simulink model "seesaw_quick_start"  (Simulink 7.8)
settings: Solver=ode1  StartTime=0.0  StopTime=inf  FixedStep=0.002  RelTol=1e-3
PostLoadFcn:
  | qc_set_target_type(getConfigSet(bdroot, 'QUARC Default Target Configuration'));
undefined symbols (not defined in the file): HIL
libraries: quarc_library x4, simulink x1
settings Model: Creator=pmartin  LastModifiedBy=pmartin  SimulationMode=external  ExtModeTrigDuration=5000
settings SolverCC: PositivePriorityOrder=on
settings OptimizationCC: InitFltsAndDblsToZero=on
settings DebuggingCC: SaveWithParameterizedLinksMsg=none  MultiTaskDSMMsg=warning  MultiTaskCondExecSysMsg=none  FcnCallInpInsideContextMsg=Use local settings  StrictBusMsg=None
settings RTWCC: SystemTargetFile=quarc_windows.tlc  TemplateMakefile=quarc_default_tmf  Description=QUARC Win32 Target  ProcessScript=quarc_windows_make_rtw_hook
settings STFCustomTargetCC: TargetPreCompLibLocation=C:\PROGRA~2\QUARC\lib\2012b\windows\release  CombineOutputUpdateFcns=on  SystemTargetFile=quarc_windows.tlc
settings GRTTargetCC: TargetPreCompLibLocation=C:\PROGRA~2\QUARC\lib\2012b\windows\release  ParMdlRefBuildCompliant=off  CompOptLevelCompliant=off  ConcurrentExecutionCompliant=off  CombineOutputUpdateFcns=on  MatFileLogging=off  ExtMode=on  ExtModeMexFile=quarc_comm

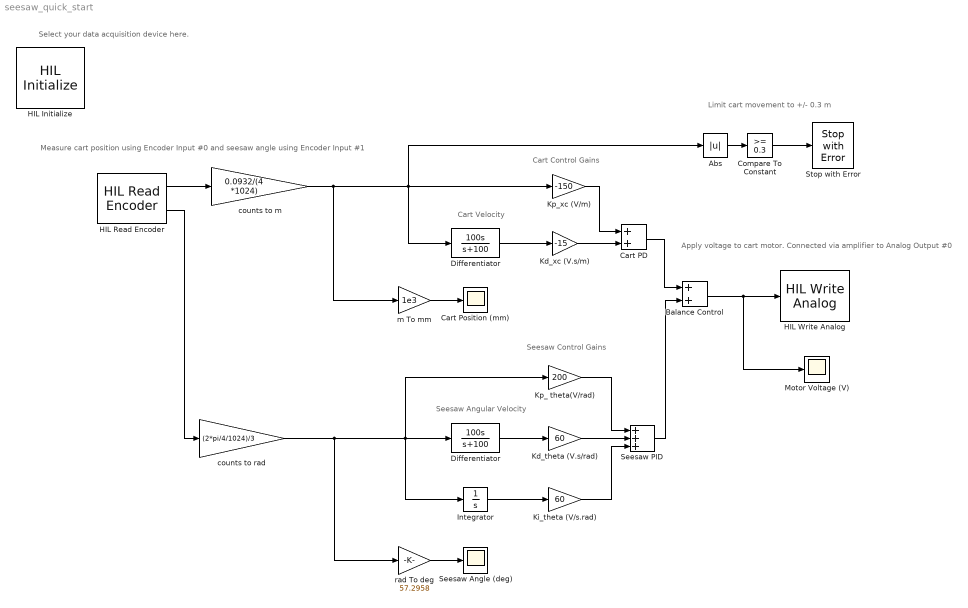
== system seesaw_quick_start ==
  note: Measure cart position using Encoder Input #0
      | and seesaw angle using Encoder Input #1
  note: Select your data acquisition device here.
  note: Cart Control Gains
  note: Cart Velocity
  note: Seesaw Angular Velocity
  note: Seesaw Control Gains
  note: Limit cart movement to +/- 0.3 m
  note: Apply voltage to cart motor.
      | Connected via amplifier to Analog Output #0
  Abs : Abs
  Balance Control : Sum
  Cart PD : Sum
  Cart Position (mm) : Scope
      settings: TickLabels=on  TimeRange=5  YMin=-25  YMax=25  SaveName=data_xc
  Compare To Constant : simulink/Logic and Bit Operations/Compare To Constant  relop=>=  const=0.3  OutDataTypeStr=boolean
  Differentiator : TransferFcn  Numerator=[100 0]  Denominator=[1 100]
  "Differentiator " : TransferFcn  Numerator=[100 0]  Denominator=[1 100]
  HIL Initialize : quarc_library/Data Acquisition/Generic/Configuration/HIL Initialize  object_name=HIL-1  board_type=q2_usb  board_number=0  board_options=d0=digital;d1=digital;led=auto;update_rate=normal  exclusive=off  active=off  hardware_clocks=[0:2]  clock_modes=[]  initial_clock_frequencies=[]  set_clock_params_at_start=off  set_clock_params_at_switch_in=off  set_clock_frequencies_at_start=off  set_clock_frequencies_at_switch_in=off  analog_input_channels=[0:1]  analog_input_maximums=10  analog_input_minimums=-10  set_analog_input_params_at_start=on  set_analog_input_params_at_switch_in=off  analog_output_channels=[0:1]  analog_output_maximums=10  analog_output_minimums=-10  initial_analog_outputs=[0]  final_analog_outputs=[0]  watchdog_analog_outputs=0  set_analog_output_params_at_start=on  set_analog_output_params_at_switch_in=off  set_analog_outputs_at_start=on  set_analog_outputs_at_switch_in=off  set_analog_outputs_at_terminate=on  set_analog_outputs_at_switch_out=off  set_analog_outputs_on_watchdog=off  digital_input_channels=[]  digital_output_channels=[0:7]  digital_output_configuration=[]  initial_digital_outputs=[0]  final_digital_outputs=[0]  watchdog_digital_outputs=[0]  set_digital_output_params_at_start=off  set_digital_output_params_at_switch_in=off  set_digital_outputs_at_start=on  set_digital_outputs_at_switch_in=off  set_digital_outputs_at_terminate=on  set_digital_outputs_at_switch_out=off  set_digital_outputs_on_watchdog=off  encoder_channels=[0:1]  quadrature=[4]  encoder_filter_frequency=[]  initial_encoder_counts=[0]  set_encoder_params_at_start=on  set_encoder_params_at_switch_in=off  set_encoder_counts_at_start=on  set_encoder_counts_at_switch_in=off  pwm_channels=[]  pwm_modes=[0]  pwm_frequency=1/0.020  pwm_configuration=[]  pwm_alignment=[]  pwm_polarity=[]  pwm_leading_deadband=[]  pwm_trailing_deadband=[]  initial_pwm_outputs=[0]  final_pwm_outputs=[0]  watchdog_pwm_outputs=[0]  set_pwm_params_at_start=on  set_pwm_params_at_switch_in=off  set_pwm_outputs_at_start=on  set_pwm_outputs_at_switch_in=off  set_pwm_outputs_at_terminate=on  set_pwm_outputs_at_switch_out=off  set_pwm_outputs_on_watchdog=off  other_output_channels=[]  initial_other_outputs=[]  final_other_outputs=[]  watchdog_other_outputs=[]  set_other_outputs_at_start=off  set_other_outputs_at_switch_in=off  set_other_outputs_at_terminate=off  set_other_outputs_at_switch_out=off  set_other_outputs_on_watchdog=off
  HIL Read Encoder : quarc_library/Data Acquisition/Generic/Immediate I//O/HIL Read Encoder  object_name=HIL-1  channels=[0:1]  sample_time=qc_get_step_size  active=on  vector_output=off  data_type_mode=Inherit via back propagation  data_type=double
  HIL Write Analog : quarc_library/Data Acquisition/Generic/Immediate I//O/HIL Write Analog  object_name=HIL-1  channels=0  sample_time=-1  active=off  vector_input=off
  Integrator : Integrator
  Kd_theta (V.s/rad) : Gain  Gain=60
  Kd_xc (V.s/m) : Gain  Gain=-15
  Ki_theta (V/s.rad) : Gain  Gain=60
  Kp_ theta(V/rad) : Gain  Gain=200
  Kp_xc (V/m) : Gain  Gain=-150
  Motor Voltage (V) : Scope
  Seesaw Angle (deg) : Scope
      settings: TimeRange=5  YMin=-32.5  YMax=32.5  SaveName=data_xjc
  Seesaw PID : Sum  Inputs=+++
  Stop with Error : quarc_library/Sinks/Error Handling/Stop with Error  message_type=Fixed error message  message=Cart position limit reached
      settings: AttributesFormatString="\"%<message>\""
  counts to m : Gain  Gain=0.0932/(4 *1024)  SaturateOnIntegerOverflow=on  OutDataTypeStr=Inherit: Same as input  ParamDataTypeStr=Inherit: Same as input
  "counts to rad " : Gain  Gain=(2*pi/4/1024)/3  SaturateOnIntegerOverflow=on  OutDataTypeStr=Inherit: Same as input  ParamDataTypeStr=Inherit: Same as input
  m To mm : Gain  Gain=1e3  SaturateOnIntegerOverflow=on  OutDataTypeStr=Inherit: Same as input  ParamDataTypeStr=Inherit: Same as input
  "rad To deg " : Gain  Gain=57.2958  SaturateOnIntegerOverflow=on  OutDataTypeStr=Inherit: Same as input  ParamDataTypeStr=Inherit: Same as input
  wires:
  HIL Read Encoder/1 -> counts to m/1
  HIL Read Encoder/2 -> "counts to rad "/1
  m To mm/1 -> Cart Position (mm)/1
  "rad To deg "/1 -> Seesaw Angle (deg)/1
  Kd_xc (V.s/m)/1 -> Cart PD/2
  Kp_xc (V/m)/1 -> Cart PD/1
  Kd_theta (V.s/rad)/1 -> Seesaw PID/2
  Kp_ theta(V/rad)/1 -> Seesaw PID/1
  Cart PD/1 -> Balance Control/1
  Seesaw PID/1 -> Balance Control/2
  Abs/1 -> Compare To Constant/1
  Balance Control/1 -> HIL Write Analog/1, Motor Voltage (V)/1
  counts to m/1 -> m To mm/1, Abs/1, Differentiator/1, Kp_xc (V/m)/1
  Differentiator/1 -> Kd_xc (V.s/m)/1
  "counts to rad "/1 -> "rad To deg "/1, Integrator/1, "Differentiator "/1, Kp_ theta(V/rad)/1
  "Differentiator "/1 -> Kd_theta (V.s/rad)/1
  Integrator/1 -> Ki_theta (V/s.rad)/1
  Ki_theta (V/s.rad)/1 -> Seesaw PID/3
  Compare To Constant/1 -> Stop with Error/1
